simulink model "FreePortComm_TX_simple"  (Simulink 7.4)
settings: Solver=FixedStepDiscrete  SolverMode=SingleTasking  StartTime=0.0  StopTime=inf  FixedStep=.02  RelTol=1e-3
settings Model: Creator=Admin  LastModifiedBy=fw  ExtModeTrigDuration=500
settings ConfigSet: Description=rtmc9s12target_R2008a
settings DataIOCC: SignalLoggingName=sigsOut
settings OptimizationCC: BooleanDataType=off  InitFltsAndDblsToZero=on
settings DebuggingCC: SaveWithParameterizedLinksMsg=none  SignalResolutionControl=TryResolveAllWithWarning  SolverPrmCheckMsg=none  MultiTaskDSMMsg=warning  MultiTaskCondExecSysMsg=none  StrictBusMsg=None
settings HardwareCC: ProdBitPerInt=16  ProdEndianess=BigEndian  ProdWordSize=16  ProdHWDeviceType=Motorola HC12  TargetHWDeviceType=32-bit Generic  ProdEqTarget=off
settings RTWCC: GenerateMakefile=off  TemplateMakefile=grt_msvc.tmf  Description="Visual C/C++ Project Makefile only for the \"grt\" target"  ProcessScript=grt_make_rtw_hook  IncludeERTFirstTime=on
settings GRTTargetCC: TargetFcnLib=ansi_tfl_tmw.mat

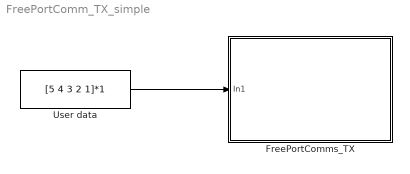
== system FreePortComm_TX_simple ==
  FreePortComms_TX : Subsystem  Tag=mcTarget_freePortCommsTX  mask{sampletime=0.1, port=COM1, baudrate=115200, channel=0, buf_size=5, data_type=UINT8, format=off}
      mask prompts: sampletime "Sample time"; port "Communication port"; channel "Channel number"; buf_size "Number of elements"; data_type "Data Type"; format "Block sends raw data"
      mask init:
      | [buf_sizestr, portNamestr, baudratestr, channelstr, data_type_str, sampletime_str] = mbc_freeporttxd(sampletime, port, baudrate, channel, buf_size, data_type, format);
      mask Help: web('freePortComms_txd.html');
      mask StyleString: edit,popup(SCI0|SCI1|COM1|COM2|COM3|COM4),popup(300|600|1200|2400|4800|9600|19200|38400|57600|115200),edit,edit,popup(SINGLE|INT8|UINT8|INT16|UINT16|INT32|UINT32|BOOLEAN),checkbox
      mask Display: fprintf('Transmit %s element(s)\nComm port: %s\nBaudrate: %s bps\nChannel: %s\nData type: %s\n Sample rate: %s', buf_sizestr, portNamestr, baudratestr, channelstr, data_type_str, sampletime_str)
  User data : Constant  Value=[5 4 3 2 1]*1  OutDataType=sfix(16)  OutScaling=2^0
  wires:
  User data/1 -> FreePortComms_TX/1(In1)

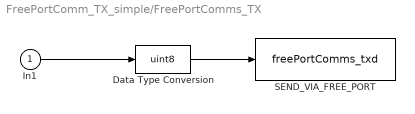
== system FreePortComm_TX_simple/FreePortComms_TX ==
  In1 : Inport  OutDataType=sfix(16)  OutScaling=2^0
  Data Type Conversion : DataTypeConversion  OutDataTypeMode=uint8  OutDataType=sfix(16)  OutScaling=2^0  OutDataTypeStr=uint8  SaturateOnIntegerOverflow=on  RndMeth=Zero
  SEND_VIA_FREE_PORT : S-Function  Tag=mcTarget_freePortCommsTX  FunctionName=freePortComms_txd  Parameters=sampletime, channel, buf_size, data_type, port, baudrate, format  EnableBusSupport=off
  wires:
  In1/1 -> Data Type Conversion/1
  Data Type Conversion/1 -> SEND_VIA_FREE_PORT/1
